simulink model "Information_Flow_Model"  (R2023b)
settings: Solver=VariableStepAuto  StartTime=0.0  StopTime=0.5  MaxStep=1e-5  RelTol=1e-3  AbsTol=1e-3  EnableMultiTasking=on
PreLoadFcn:
  | m = 3.600;     % kg
  | k = 400;    % N/m
  | b = 10;      % Ns/m
  | x0=1; %m
values from neighbouring files (symbols this model uses):
  mems_b = b1+b2    (= 0.000950957529895)    [System_Analytics.m]
  mems_k = 2*((pi^4 / 6) * (E_silicon * t * w_s^3 / ((2*L_s1)^3+(2*L_s1)^3)))    (= 68.9981061491)    [System_Analytics.m]
  mems_mass = (calculate_proof_mass(length_m, width, thickness, density_si, N, comb_l,comb_w))    [System_Analytics.m]
CloseFcn:
  | try,close(h1_MassSpringDamperInSimulinkAndSimscape),end
  | clear h1_MassSpringDamperInSimulinkAndSimscape
  | 
  | clear simlog_MassSpringDamperInSimulinkAndSimscape
  | clear logsout_MassSpringDamperInSimulinkAndSimscape
Description:
  | Mass-Spring-Damper in Simulink(R) and Simscape(TM)
settings Model: Creator=The MathWorks, Inc.  LastModifiedBy=241pr
settings SolverCC: AutoScaleAbsTol=off  AlgebraicLoopSolver=TrustRegion
settings DataIOCC: LimitDataPoints=on  SaveFormat=Array  ReturnWorkspaceOutputs=off  SignalLoggingName=logsout_MassSpringDamperInSimulinkAndSimscape
settings OptimizationCC: LifeSpan=inf
settings DebuggingCC: SolverPrmCheckMsg=warning  UnconnectedInputMsg=warning  UnconnectedOutputMsg=warning  UnconnectedLineMsg=warning  AllowSymbolicDim=off  PregeneratedLibrarySubsystemCodeDiagnostic=none  SFUnexpectedBacktrackingDiag=warning  SFNoUnconditionalDefaultTransitionDiag=warning  SFExecutionAtInitializationDiag=none  ArithmeticOperatorsInVariantConditions=warning
settings HardwareCC: ProdBitPerPointer=32  ProdBitPerSizeT=32  ProdBitPerPtrDiffT=32  ProdLargestAtomicFloat=None  ProdIntDivRoundTo=Undefined  ProdEndianess=Unspecified  ProdWordSize=32  ProdHWDeviceType=32-bit Generic
settings ModelReferenceCC: EnableRefExpFcnMdlSchedulingChecks=on  PropagateSignalLabelsOutOfModel=off
settings SFSimCC: SimUseLocalCustomCode=off  CustomCodeUndefinedFunction=UseInterfaceOnly
settings RTWCC: RTWUseLocalCustomCode=off  DLArmComputeVersion=19.05
settings CodeAppCC: StateflowObjectComments=on
settings GRTTargetCC: TargetLangStandard=C89/C90 (ANSI)
settings ConfigComp: CovMetricSettings=dw  CovSaveCumulativeToWorkspaceVar=on  CovSaveSingleToWorkspaceVar=on  CovExternalEMLEnable=off  CovSFcnEnable=off
settings SimscapeCC: SimscapeLogType=all  SimscapeLogSimulationStatistics=on  SimscapeLogName=simlog_MassSpringDamperInSimulinkAndSimscape  SimscapeLogDataHistory=10000

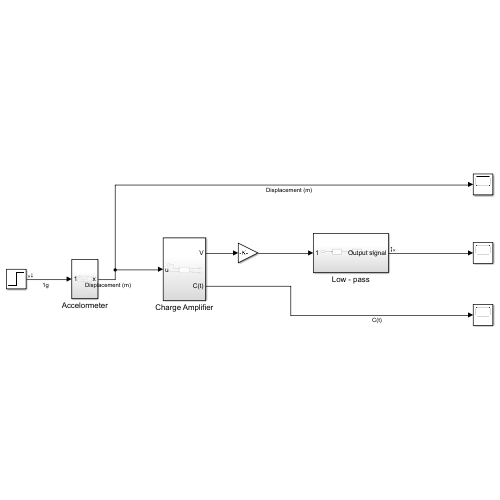
[thumbnail: Simulink's stored preview of the top-level diagram]
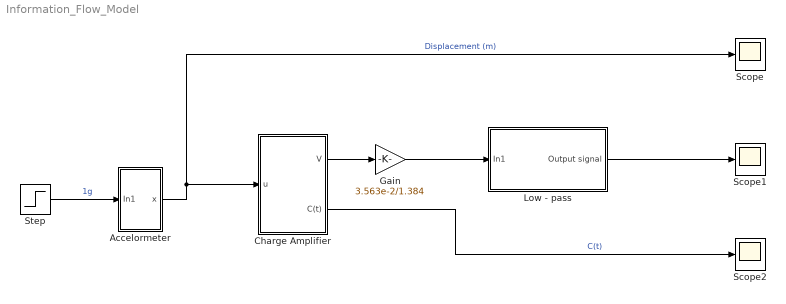
== system Information_Flow_Model ==
  Accelormeter : Subsystem
  Charge Amplifier : Subsystem
  Gain : Gain  Gain=3.563e-2/1.384
  Low - pass : Subsystem
  Scope : Scope
  Scope1 : Scope
  Scope2 : Scope
  Step : Step  Time=0.1  After=9.81*mems_mass  SampleTime=0
  wires:
  Accelormeter/1(x) -> Scope/1, Charge Amplifier/1(u)  "Displacement (m)"
  Step/1 -> Accelormeter/1(In1)  "1g"
  Charge Amplifier/1(V) -> Gain/1
  Charge Amplifier/2(C(t)) -> Scope2/1  "C(t)"
  Gain/1 -> Low - pass/1(In1)
  Low - pass/1(Output signal) -> Scope1/1

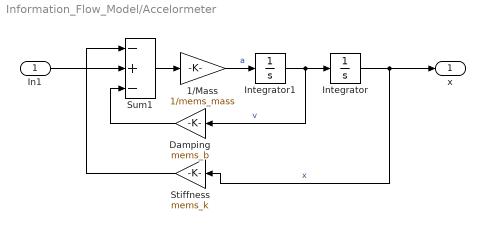
== system Information_Flow_Model/Accelormeter ==
  In1 : Inport
  "1/Mass " : Gain  Gain=1/mems_mass  SaturateOnIntegerOverflow=on  OutDataTypeStr=Inherit: Same as input  ParamDataTypeStr=Inherit: Same as input
  Damping : Gain  Gain=mems_b  SaturateOnIntegerOverflow=on  OutDataTypeStr=Inherit: Same as input  ParamDataTypeStr=Inherit: Same as input
  Integrator : Integrator
  Integrator1 : Integrator
  Stiffness : Gain  Gain=mems_k  SaturateOnIntegerOverflow=on  OutDataTypeStr=Inherit: Same as input  ParamDataTypeStr=Inherit: Same as input
  Sum1 : Sum  Inputs=-+-  InputSameDT=on  SaturateOnIntegerOverflow=on  OutDataTypeStr=Inherit: Same as first input
  x : Outport
  wires:
  Sum1/1 -> "1/Mass "/1
  "1/Mass "/1 -> Integrator1/1  "a"
  Stiffness/1 -> Sum1/1
  Integrator/1 -> x/1, Stiffness/1  "x"
  Damping/1 -> Sum1/3
  In1/1 -> Sum1/2
  Integrator1/1 -> Integrator/1, Damping/1  "v"

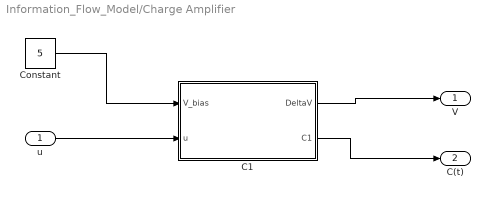
== system Information_Flow_Model/Charge Amplifier ==
  u : Inport
  C1 : MATLAB Function  TreatAsAtomicUnit=on
  Constant : Constant  Value=5
  V : Outport
  C(t) : Outport  Port=2
  wires:
  u/1 -> C1/2(u)
  C1/1(DeltaV) -> V/1
  C1/2(C1) -> C(t)/1
  Constant/1 -> C1/1(V_bias)

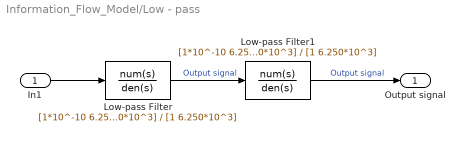
== system Information_Flow_Model/Low - pass ==
  In1 : Inport
  Low-pass Filter : TransferFcn  Numerator=[1*10^-10 6.250*10^3]  Denominator=[1 6.250*10^3]
  Low-pass Filter1 : TransferFcn  Numerator=[1*10^-10 6.250*10^3]  Denominator=[1 6.250*10^3]
  Output signal : Outport
  wires:
  Low-pass Filter/1 -> Low-pass Filter1/1  "Output signal"
  Low-pass Filter1/1 -> Output signal/1  "Output signal"
  In1/1 -> Low-pass Filter/1

== matlab function Information_Flow_Model/Charge Amplifier/C1 ==
  data: V_bias input; u input; DeltaV output; C1 output

function [DeltaV, C1] = DeltaV(V_bias,u)

N=70;
e=8.854e-12;
t=25e-6;
l=810e-6;
d1=10e-6;
C2=(e*N*l*t/(d1))*(1-u/d1);
C1 = (e*N*l*t/(d1))*(1+u/d1); 

DeltaV = (V_bias*((C1-C2)/(5.95e-14))) ;
